simulink model "spring_system"  (R2015a)
settings: Solver=ode45  StartTime=0.0  StopTime=4  MaxStep=1/60  RelTol=1e-3
settings Model: Creator=Anıl  LastModifiedBy=Anıl

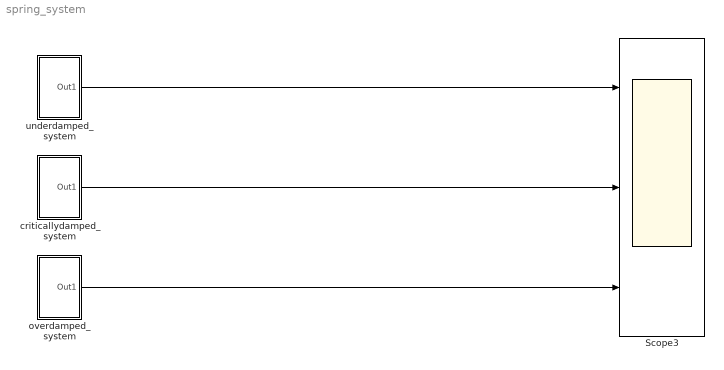
== system spring_system ==
  Scope3 : Scope  NumInputPorts=3
      settings: YMin=-5~-5~-5  YMax=5~5~5  SaveName=ScopeData3
  criticallydamped_system : Subsystem
  "overdamped_system " : Subsystem
  underdamped_system : Subsystem
  wires:
  underdamped_system/1(Out1) -> Scope3/1
  criticallydamped_system/1(Out1) -> Scope3/2
  "overdamped_system "/1(Out1) -> Scope3/3

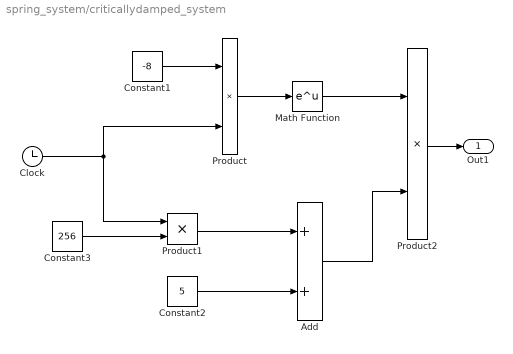
== system spring_system/criticallydamped_system ==
  Add : Sum
  Clock : Clock
  Constant1 : Constant  Value=-8
  Constant2 : Constant  Value=5
  Constant3 : Constant  Value=256
  Math Function : Math  SaturateOnIntegerOverflow=on
  Product : Product
  Product1 : Product
  Product2 : Product
  Out1 : Outport
  wires:
  Product2/1 -> Out1/1
  Math Function/1 -> Product2/1
  Constant1/1 -> Product/1
  Constant3/1 -> Product1/2
  Clock/1 -> Product/2, Product1/1
  Product/1 -> Math Function/1
  Add/1 -> Product2/2
  Constant2/1 -> Add/2
  Product1/1 -> Add/1

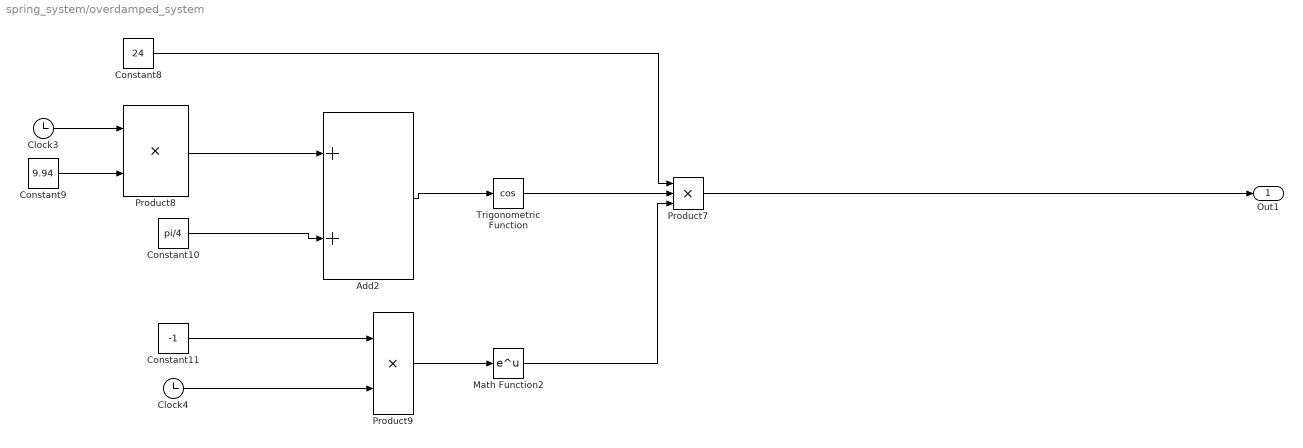
== system spring_system/overdamped_system  ==
  Add2 : Sum
  Clock3 : Clock
  Clock4 : Clock
  Constant10 : Constant  Value=pi/4
  Constant11 : Constant  Value=-1
  Constant8 : Constant  Value=24
  Constant9 : Constant  Value=9.94
  Math Function2 : Math  SaturateOnIntegerOverflow=on
  Product7 : Product  Inputs=3
  Product8 : Product
  Product9 : Product
  Trigonometric Function : Trigonometry  Operator=cos
  Out1 : Outport
  wires:
  Product9/1 -> Math Function2/1
  Product7/1 -> Out1/1
  Clock4/1 -> Product9/2
  Trigonometric Function/1 -> Product7/2
  Constant11/1 -> Product9/1
  Add2/1 -> Trigonometric Function/1
  Constant8/1 -> Product7/1
  Clock3/1 -> Product8/1
  Constant9/1 -> Product8/2
  Math Function2/1 -> Product7/3
  Constant10/1 -> Add2/2
  Product8/1 -> Add2/1

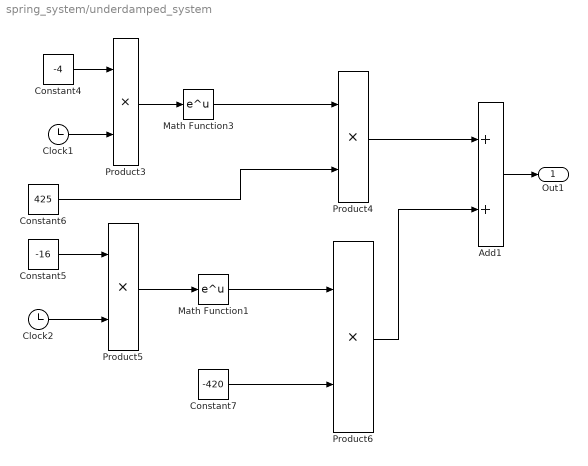
== system spring_system/underdamped_system ==
  Add1 : Sum
  Clock1 : Clock
  Clock2 : Clock
  Constant4 : Constant  Value=-4
  Constant5 : Constant  Value=-16
  Constant6 : Constant  Value=425
  Constant7 : Constant  Value=-420
  Math Function1 : Math  SaturateOnIntegerOverflow=on
  Math Function3 : Math  SaturateOnIntegerOverflow=on
  Product{3..6} (4 alike) : Product
  Out1 : Outport
  wires:
  Constant6/1 -> Product4/2
  Clock2/1 -> Product5/2
  Constant5/1 -> Product5/1
  Product5/1 -> Math Function1/1
  Math Function1/1 -> Product6/1
  Constant7/1 -> Product6/2
  Add1/1 -> Out1/1
  Product6/1 -> Add1/2
  Product4/1 -> Add1/1
  Clock1/1 -> Product3/2
  Product3/1 -> Math Function3/1
  Math Function3/1 -> Product4/1
  Constant4/1 -> Product3/1
